simulink model "bpsk_receiver"  (R2020a)
settings: Solver=VariableStepAuto  StartTime=0.0  StopTime=10000/3.2e6  RelTol=1e-3
InitFcn:
  | setup_bpsk_receiver
undefined symbols (not defined in the file): AXI4, designMultirateFIR, fir_bbuf, Lite, tx_data, xlfda_numerator
libraries: xbsIndex_r4 x367, hdlsllib x15, dspmlti4 x8, xrbsSSR_Library x6, dspswit3 x4, dspsigops x2, commrandsrc3 x1, simulink x1
(part 2 of 4)

== system bpsk_receiver/Frame Synchronisation ==
  Reset : Inport
  Threshold : Inport  Port=2
  Valid In : Inport  Port=3
  Real In : Inport  Port=4
  Convert to AXI-Stream : Subsystem
  Frame Sync : Subsystem
  Valid Out : Outport  VectorParamsAs1DForOutWhenUnconnected=off
  Data Out : Outport  Port=2  VectorParamsAs1DForOutWhenUnconnected=off
  Last Out : Outport  Port=3  VectorParamsAs1DForOutWhenUnconnected=off
  Size : Outport  Port=4  VectorParamsAs1DForOutWhenUnconnected=off
  Count : Outport  Port=5  VectorParamsAs1DForOutWhenUnconnected=off
  wires:
  Convert to AXI-Stream/4(Size) -> Size/1
  Frame Sync/3(count) -> Count/1
  Convert to AXI-Stream/5(Reset) -> Frame Sync/5(Reset)
  Convert to AXI-Stream/3(Last Out) -> Last Out/1
  Convert to AXI-Stream/2(Valid Out) -> Valid Out/1
  Convert to AXI-Stream/1(Data Out) -> Data Out/1
  Frame Sync/2(Valid Out) -> Convert to AXI-Stream/2(Valid In)
  Frame Sync/1(Data Out) -> Convert to AXI-Stream/1(Data In)
  Reset/1 -> Frame Sync/4(reset_count)
  Valid In/1 -> Frame Sync/3(Valid In)
  Real In/1 -> Frame Sync/2(Data In)
  Threshold/1 -> Frame Sync/1(Threshold)

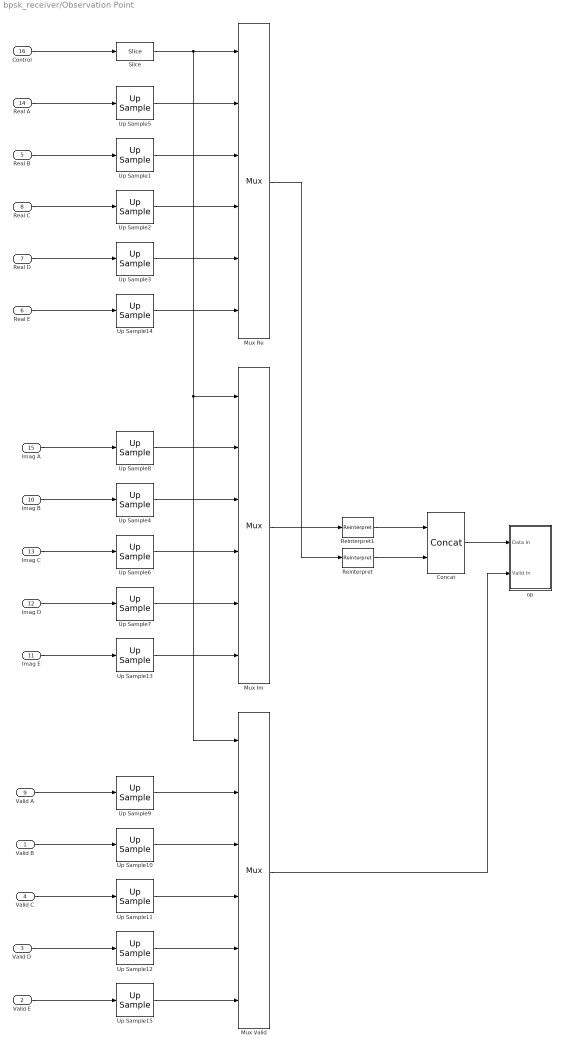
== system bpsk_receiver/Observation Point ==
  Valid B : Inport
  Valid E : Inport  Port=2
  Valid D : Inport  Port=3
  Valid C : Inport  Port=4
  Real B : Inport  Port=5
  Real E : Inport  Port=6
  Real D : Inport  Port=7
  Real C : Inport  Port=8
  Valid A : Inport  Port=9
  Imag B : Inport  Port=10
  Imag E : Inport  Port=11
  Imag D : Inport  Port=12
  Imag C : Inport  Port=13
  Real A : Inport  Port=14
  Imag A : Inport  Port=15
  Control : Inport  Port=16
  Concat : xbsIndex_r4/Concat  num_inputs=2  dbl_ovrd=off  block_type=concat
  Mux Im : xbsIndex_r4/Mux  inputs=5  en=off  latency=1  precision=Full  arith_type=Unsigned  n_bits=16  bin_pt=14  quantization=Truncate  overflow=Wrap  dbl_ovrd=off  block_type=mux
  Mux Re : xbsIndex_r4/Mux  inputs=5  en=off  latency=1  precision=Full  arith_type=Unsigned  n_bits=16  bin_pt=14  quantization=Truncate  overflow=Wrap  dbl_ovrd=off  block_type=mux
  Mux Valid : xbsIndex_r4/Mux  inputs=5  en=off  latency=1  precision=Full  arith_type=Unsigned  n_bits=16  bin_pt=14  quantization=Truncate  overflow=Wrap  dbl_ovrd=off  block_type=mux
  Reinterpret : xbsIndex_r4/Reinterpret  force_arith_type=on  arith_type=Unsigned  force_bin_pt=on  bin_pt=0  block_type=reinterpret
  Reinterpret1 : xbsIndex_r4/Reinterpret  force_arith_type=on  arith_type=Unsigned  force_bin_pt=on  bin_pt=0  block_type=reinterpret
  Slice : xbsIndex_r4/Slice  nbits=1  boolean_output=off  mode=Two Bit Locations  bit1=2  base1=LSB of Input  bit0=0  base0=LSB of Input  dbl_ovrd=off  block_type=slice
  Up Sample{1..2,4..6,8} (6 alike) : xbsIndex_r4/Up Sample  sample_ratio=64e6/3.2e6  copy_samples=on  en=off  latency=0  dbl_ovrd=off  block_type=usamp
  Up Sample10 : xbsIndex_r4/Up Sample  sample_ratio=64e6/3.2e6  copy_samples=off  en=off  latency=0  dbl_ovrd=off  block_type=usamp
  Up Sample11 : xbsIndex_r4/Up Sample  sample_ratio=64e6/3.2e6  copy_samples=off  en=off  latency=0  dbl_ovrd=off  block_type=usamp
  Up Sample12 : xbsIndex_r4/Up Sample  sample_ratio=64e6/12.8e6  copy_samples=off  en=off  latency=0  dbl_ovrd=off  block_type=usamp
  Up Sample{3,7,13..14} (4 alike) : xbsIndex_r4/Up Sample  sample_ratio=64e6/12.8e6  copy_samples=on  en=off  latency=0  dbl_ovrd=off  block_type=usamp
  Up Sample15 : xbsIndex_r4/Up Sample  sample_ratio=64e6/12.8e6  copy_samples=off  en=off  latency=0  dbl_ovrd=off  block_type=usamp
  Up Sample9 : xbsIndex_r4/Up Sample  sample_ratio=64e6/3.2e6  copy_samples=off  en=off  latency=0  dbl_ovrd=off  block_type=usamp
  op : Subsystem
  wires:
  Valid B/1 -> Up Sample10/1
  Up Sample10/1 -> Mux Valid/3
  Control/1 -> Slice/1
  Up Sample1/1 -> Mux Re/3
  Concat/1 -> op/1(Data In)
  Mux Re/1 -> Reinterpret/1
  Real B/1 -> Up Sample1/1
  Up Sample11/1 -> Mux Valid/4
  Up Sample2/1 -> Mux Re/4
  Mux Valid/1 -> op/2(Valid In)
  Up Sample3/1 -> Mux Re/5
  Up Sample6/1 -> Mux Im/4
  Up Sample12/1 -> Mux Valid/5
  Imag A/1 -> Up Sample8/1
  Real A/1 -> Up Sample5/1
  Reinterpret/1 -> Concat/2
  Up Sample7/1 -> Mux Im/5
  Reinterpret1/1 -> Concat/1
  Imag C/1 -> Up Sample6/1
  Up Sample5/1 -> Mux Re/2
  Up Sample4/1 -> Mux Im/3
  Up Sample8/1 -> Mux Im/2
  Mux Im/1 -> Reinterpret1/1
  Up Sample9/1 -> Mux Valid/2
  Valid A/1 -> Up Sample9/1
  Imag D/1 -> Up Sample7/1
  Valid D/1 -> Up Sample12/1
  Real D/1 -> Up Sample3/1
  Valid C/1 -> Up Sample11/1
  Valid E/1 -> Up Sample15/1
  Imag E/1 -> Up Sample13/1
  Real C/1 -> Up Sample2/1
  Imag B/1 -> Up Sample4/1
  Real E/1 -> Up Sample14/1
  Slice/1 -> Mux Valid/1, Mux Im/1, Mux Re/1
  Up Sample13/1 -> Mux Im/6
  Up Sample14/1 -> Mux Re/6
  Up Sample15/1 -> Mux Valid/6

== system bpsk_receiver/RRC Receive Filter ==
  Valid In : Inport
  Real In : Inport  Port=2
  Imag In : Inport  Port=3
  Convert : xbsIndex_r4/Convert  gui_display_data_type=Fixed-point  arith_type="Signed  (2's comp)"  n_bits=16  bin_pt=14  float_type=Single  exp_bits=8  fraction_bits=24  quantization=Truncate  overflow=Wrap  en=off  latency=0  pipeline=off  dbl_ovrd=off  block_type=convert
  Convert1 : xbsIndex_r4/Convert  gui_display_data_type=Fixed-point  arith_type="Signed  (2's comp)"  n_bits=16  bin_pt=14  float_type=Single  exp_bits=8  fraction_bits=24  quantization=Truncate  overflow=Wrap  en=off  latency=0  pipeline=off  dbl_ovrd=off  block_type=convert
  FDATool : xbsIndex_r4/FDATool  block_type=fdatool
      settings: infoedit=FDATool
  "FIR Compiler 7.2 " : xbsIndex_r4/FIR Compiler 7.2   coefficientvector=xlfda_numerator('FDATool')  coefficient_sets=1  coefficient_reload=off  filter_type=Decimation  rate_change_type=Integer  interpolation_rate=1  decimation_rate=4  zero_pack_factor=1  channel_sequence=Basic  number_channels=1  pattern_list='P4-0,P4-1,P4-2,P4-3,P4-4'  number_paths=2  ratespecification=Maximum_Possible  sampleperiod=1  hardwareoversamplingrate=1  coefficient_sign=Signed  quantization=Quantize_Only  coefficient_width=16  bestprecision=on  coefficient_fractional_bits=16  coefficient_structure=Inferred  output_rounding_mode=Full_Precision  output_width=33  filter_architecture=Systolic_Multiply_Accumulate  optimization_goal=Area  optimization_list='None'  data_buffer_type=Automatic  coefficient_buffer_type=Automatic  input_buffer_type=Automatic  output_buffer_type=Automatic  preference_for_other_storage=Automatic  multi_column_support=Automatic  columnconfig='6'  inter_column_pipe_length=4  data_has_tlast=Not_Required  m_data_has_tready=off  s_data_has_fifo=off  s_data_has_tuser=Not_Required  m_data_has_tuser=Not_Required  s_config_sync_mode=On_Vector  s_config_method=Single  num_reload_slots=1  has_aclken=off  has_aresetn=off  infoeditControl=ARESETn must be asserted for a minimum of 2 cycles  reset_data_vector=on  trim_axipin_name=on  simulation_type=hybrid_sim  simulation_model=sysgen:xfirv7_2_cmodel  data_path_portlist={ 's_axis_data_tdata', 'm_axis_data_tdata' }  passband_min=0.0  passband_max=0.5  stopband_min=0.5  stopband_max=1.0  filter_selection=1  gui_behaviour='Sysgen_GUI'  data_sign=Signed  data_width=16  data_fractional_bits=0  data_tuser_width=1  wrapper_available=true  ip_wrap_arbitrary_binary_point=true  ip_name=FIR Compiler  ip_version=7.2  dsptool_ready=true  ipcore_usecache=true  ipcore_useipmodelcache=true  port_translation_map={ 'aclken' => 'en', 'aresetn' => 'rst' }  run_core_at_system_period=true  ipcore_xco_need_fpga_part=true  block_type=fir_compiler_v7_2
      settings: infoedit=Maximum Possible : Maximizes oversampling rate. Abstracted input handshake (no s_data_tvalid) and automatic rate propagation.<br>Hardware Oversampling Rate : Specifies oversampling rate relative to the input sample period. Abstracted input handshake (no s_data_tvalid) and automatic rate propagation.<br>Input/Output Sample Period : Specifies absolute oversampling rate. No input handshake abstraction (exposes s_data_tvalid) and no rate propagation.
  Terminator2 : Terminator
  Terminator4 : Terminator
  Valid Out : Outport  VectorParamsAs1DForOutWhenUnconnected=off
  Real Out : Outport  Port=2  VectorParamsAs1DForOutWhenUnconnected=off
  Imag Out : Outport  Port=3  VectorParamsAs1DForOutWhenUnconnected=off
  wires:
  "FIR Compiler 7.2 "/2 -> Valid Out/1
  "FIR Compiler 7.2 "/4 -> Convert1/1
  Imag In/1 -> "FIR Compiler 7.2 "/2
  "FIR Compiler 7.2 "/1 -> Terminator2/1
  Real In/1 -> "FIR Compiler 7.2 "/1
  Convert/1 -> Real Out/1
  "FIR Compiler 7.2 "/3 -> Convert/1
  Convert1/1 -> Imag Out/1
  Valid In/1 -> Terminator4/1

== system bpsk_receiver/SSR Halfband Lowpass Decimator ==
  Valid In : Inport
  Real In : Inport  Port=2
  Imag In : Inport  Port=3
  Convert : xbsIndex_r4/Convert  gui_display_data_type=Fixed-point  arith_type="Signed  (2's comp)"  n_bits=16  bin_pt=14  float_type=Single  exp_bits=8  fraction_bits=24  quantization="Round  (unbiased: +/- Inf)"  overflow=Saturate  en=off  latency=0  pipeline=off  dbl_ovrd=off  block_type=convert
  Convert1 : xbsIndex_r4/Convert  gui_display_data_type=Fixed-point  arith_type="Signed  (2's comp)"  n_bits=16  bin_pt=14  float_type=Single  exp_bits=8  fraction_bits=24  quantization="Round  (unbiased: +/- Inf)"  overflow=Saturate  en=off  latency=0  pipeline=off  dbl_ovrd=off  block_type=convert
  FDATool : xbsIndex_r4/FDATool  block_type=fdatool
      settings: infoedit=FDATool
  Terminator1 : Terminator
  Terminator2 : Terminator
  Vector FIR Im : xrbsSSR_Library/Vector FIR  coefficientvector=xlfda_numerator('FDATool')/(max(xlfda_numerator('FDATool'))*2)  coefficient_sets=1  coeffsets_prev=1  coefficient_reload=off  filter_type=Decimation  filter_prev=Decimation  interpolation_rate=2  interpolation_prev=2  rate_change_type=Integer  decimation_rate=2  decimation_prev=2  zero_pack_factor=2  channel_sequence=Basic  number_channels=1  pattern_list='P4-0,P4-1,P4-2,P4-3,P4-4'  number_paths=1  sg_ssr=2  coefficient_sign=Signed  quantization=Quantize_Only  coefficient_width=16  bestprecision=off  coefficient_fractional_bits=14  coefficient_structure=Inferred  output_rounding_mode=Full_Precision  output_width=24  filter_architecture=Systolic_Multiply_Accumulate  optimization_goal=Area  optimization_list='None'  data_buffer_type=Automatic  coefficient_buffer_type=Automatic  input_buffer_type=Automatic  output_buffer_type=Automatic  preference_for_other_storage=Automatic  multi_column_support=Automatic  columnconfig='11'  inter_column_pipe_length=4  data_has_tlast=Not_Required  m_data_has_tready=off  s_data_has_fifo=off  s_data_has_tuser=Not_Required  m_data_has_tuser=Not_Required  s_config_sync_mode=On_Vector  s_config_method=Single  num_reload_slots=1  has_aclken=off  has_aresetn=off  infoeditControl=ARESETn must be asserted for a minimum of 2 cycles  reset_data_vector=on  simulation_type=xsim  simulation_model=sysgen:xfirv7_2_cmodel  data_path_portlist={ 's_axis_data_tdata', 'm_axis_data_tdata' }  passband_min=0.0  passband_max=0.5  stopband_min=0.5  stopband_max=1.0  filter_selection=1  gui_behaviour=1  data_sign=Signed  data_width=16  data_fractional_bits=0  data_tuser_width='11'  wrapper_available=true  ip_wrap_arbitrary_binary_point=true  ip_name=FIR Compiler  ip_version=7.2  dsptool_ready=true  ipcore_usecache=true  ipcore_useipmodelcache=true  port_translation_map={ 'aclken' => 'en', 'aresetn' => 'rst' }  run_core_at_system_period=true  ipcore_xco_need_fpga_part=true  ipcore_fpga_part=[]  block_type=fir_compiler_v7_2_ssr  sg_ssr_name=vect_FIR  sg_ssr_prev=2
      settings: SourceProductName=Xilinx SSR Blockset
  Vector FIR Re : xrbsSSR_Library/Vector FIR  coefficientvector=xlfda_numerator('FDATool')/(max(xlfda_numerator('FDATool'))*2)  coefficient_sets=1  coeffsets_prev=1  coefficient_reload=off  filter_type=Decimation  filter_prev=Decimation  interpolation_rate=2  interpolation_prev=2  rate_change_type=Integer  decimation_rate=2  decimation_prev=2  zero_pack_factor=2  channel_sequence=Basic  number_channels=1  pattern_list='P4-0,P4-1,P4-2,P4-3,P4-4'  number_paths=1  sg_ssr=2  coefficient_sign=Signed  quantization=Quantize_Only  coefficient_width=16  bestprecision=off  coefficient_fractional_bits=14  coefficient_structure=Inferred  output_rounding_mode=Full_Precision  output_width=24  filter_architecture=Systolic_Multiply_Accumulate  optimization_goal=Area  optimization_list='None'  data_buffer_type=Automatic  coefficient_buffer_type=Automatic  input_buffer_type=Automatic  output_buffer_type=Automatic  preference_for_other_storage=Automatic  multi_column_support=Automatic  columnconfig='11'  inter_column_pipe_length=4  data_has_tlast=Not_Required  m_data_has_tready=off  s_data_has_fifo=off  s_data_has_tuser=Not_Required  m_data_has_tuser=Not_Required  s_config_sync_mode=On_Vector  s_config_method=Single  num_reload_slots=1  has_aclken=off  has_aresetn=off  infoeditControl=ARESETn must be asserted for a minimum of 2 cycles  reset_data_vector=on  simulation_type=xsim  simulation_model=sysgen:xfirv7_2_cmodel  data_path_portlist={ 's_axis_data_tdata', 'm_axis_data_tdata' }  passband_min=0.0  passband_max=0.5  stopband_min=0.5  stopband_max=1.0  filter_selection=1  gui_behaviour=1  data_sign=Signed  data_width=16  data_fractional_bits=0  data_tuser_width='11'  wrapper_available=true  ip_wrap_arbitrary_binary_point=true  ip_name=FIR Compiler  ip_version=7.2  dsptool_ready=true  ipcore_usecache=true  ipcore_useipmodelcache=true  port_translation_map={ 'aclken' => 'en', 'aresetn' => 'rst' }  run_core_at_system_period=true  ipcore_xco_need_fpga_part=true  ipcore_fpga_part=[]  block_type=fir_compiler_v7_2_ssr  sg_ssr_name=vect_FIR  sg_ssr_prev=2
      settings: SourceProductName=Xilinx SSR Blockset
  Valid Out : Outport  VectorParamsAs1DForOutWhenUnconnected=off
  Real Out : Outport  Port=2  VectorParamsAs1DForOutWhenUnconnected=off
  Imag Out : Outport  Port=3  VectorParamsAs1DForOutWhenUnconnected=off
  Ready Out : Outport  Port=4  VectorParamsAs1DForOutWhenUnconnected=off
  wires:
  Convert1/1 -> Imag Out/1
  Convert/1 -> Real Out/1
  Vector FIR Im/2 -> Terminator2/1
  Vector FIR Re/1 -> Ready Out/1
  Vector FIR Im/1 -> Terminator1/1
  Vector FIR Im/3 -> Convert1/1
  Vector FIR Re/3 -> Convert/1
  Real In/1 -> Vector FIR Re/2
  Vector FIR Re/2 -> Valid Out/1
  Valid In/1 -> Vector FIR Re/1, Vector FIR Im/1
  Imag In/1 -> Vector FIR Im/2

== system bpsk_receiver/Time Synchronisation ==
  Reset : Inport
  Valid In : Inport  Port=2
  Real In : Inport  Port=3
  Imag In : Inport  Port=4
  Loop Filter : Subsystem  mask{T=1/100e3, d=1/sqrt(2), Kp=3.2, Bn=100e3*0.05, Ko=1}
      mask prompts: T "Sampling Period:"; d "Damping Ratio:"; Kp "Phase Detector Gain:"; Bn "Noise Bandwidth:"; Ko "Oscillator Gain:"
      mask init:
      | n = (Bn*T)/(d+1/(4*d));
      | 
      | K1 = ((4*d*n)/(1+2*d*n+n^2))/(Ko*Kp);
      | 
      | K2 = ((4*n^2)/(1+2*d*n+n^2))/(Ko*Kp);
      | 
      | %K1 = (4*d*n)/(Ko*Kp);
      | 
      | %K2 = (4*(n^2))/(Ko*Kp);
      mask DialogControl DescGroupVar Prompt: Loop Filter
      mask DialogControl DescTextVar Prompt: A simplified loop filter.
      mask DialogControl ParameterGroupVar Prompt: Main
  NCC : Subsystem  mask{r=32, f=58}
      mask prompts: r "Symbol Oversample Factor:"; f "Fractional Bits:"
      mask init:
      | n = ceil(log2(r))+1;
      mask DialogControl DescGroupVar Prompt: Numerically Controlled Clock (NCC)
      mask DialogControl DescTextVar Prompt: The NCC block contains an accumulator that increments by one each clock cycle. The wordlength of the accumulator is determined by the symbol oversampling factor. Once the maximum value of the accumulator is reached, the accumulation starts again. The error signal can be used to increase or decrease the rate of accumulation. When the accumulator wraps around, a binary high is released from the strobe port.
      mask DialogControl ParameterGroupVar Prompt: Main
  Terminator : Terminator
  Timing Error Detector : Subsystem
  Valid Out : Outport  VectorParamsAs1DForOutWhenUnconnected=off
  Real Out : Outport  Port=2  VectorParamsAs1DForOutWhenUnconnected=off
  Imag Out : Outport  Port=3  VectorParamsAs1DForOutWhenUnconnected=off
  wires:
  Valid In/1 -> Terminator/1
  Real In/1 -> Timing Error Detector/1(Real In), Loop Filter/1(Real In)
  Loop Filter/4(Error Out) -> NCC/1(Error)
  Timing Error Detector/1(Error) -> Loop Filter/3(Signal In)
  Imag In/1 -> Loop Filter/2(Imag In), Timing Error Detector/2(Imag In)
  Loop Filter/3(Valid Out) -> Valid Out/1
  Loop Filter/1(Real Out) -> Real Out/1
  Loop Filter/2(Imag Out) -> Imag Out/1
  NCC/1(Strobe) -> Loop Filter/4(Valid In)
  Reset/1 -> Loop Filter/5(Reset)

== system bpsk_receiver/AXI-Stream Master Interface/Rising Edge Detector Enable ==
  Input : Inport
  Inverter2 : xbsIndex_r4/Inverter  en=off  latency=0  dbl_ovrd=off  block_type=inv
  Logical3 : xbsIndex_r4/Logical  logical_function=AND  inputs=2  en=off  latency=0  precision=Full  arith_type=Unsigned  n_bits=16  bin_pt=0  align_bp=on  dbl_ovrd=off  block_type=logical
  Register1 : xbsIndex_r4/Register  init=0  rst=off  en=off  dbl_ovrd=off  block_type=register
  Output : Outport  VectorParamsAs1DForOutWhenUnconnected=off
  wires:
  Input/1 -> Logical3/2, Inverter2/1
  Inverter2/1 -> Register1/1
  Logical3/1 -> Output/1
  Register1/1 -> Logical3/1

== system bpsk_receiver/AXI-Stream Master Interface/Rising Edge Detector Last ==
  Input : Inport
  Inverter2 : xbsIndex_r4/Inverter  en=off  latency=0  dbl_ovrd=off  block_type=inv
  Logical3 : xbsIndex_r4/Logical  logical_function=AND  inputs=2  en=off  latency=0  precision=Full  arith_type=Unsigned  n_bits=16  bin_pt=0  align_bp=on  dbl_ovrd=off  block_type=logical
  Register1 : xbsIndex_r4/Register  init=0  rst=off  en=off  dbl_ovrd=off  block_type=register
  Output : Outport  VectorParamsAs1DForOutWhenUnconnected=off
  wires:
  Register1/1 -> Logical3/1
  Logical3/1 -> Output/1
  Inverter2/1 -> Register1/1
  Input/1 -> Inverter2/1, Logical3/2

== system bpsk_receiver/BPSK System/BPSK TX Generation ==
  Enable : Inport
  Bernoulli Binary Generator : commrandsrc3/Bernoulli Binary Generator  ProbabilityOfZero=0.5  SeedSource=Auto  Seed=0  SampleTime=1/100e3  SamplesPerFrame=1  OutputDataType=double  SimulateUsing=Interpreted execution
  CIC Interpolation : dspmlti4/CIC Interpolation  filtFrom=Dialog parameters  filtobj=Hm_interp  ftype=Interpolator  R=320  M=1  N=5  filterInternals=Full precision  BPS=[16 16 16 16]  FLPS=0  outputWordLength=32  outputFracLength=0  launchFVT=off  framing=Allow multirate processing  OutputFrames=off
      settings: SourceProductBaseCode=DS
  Constant : Constant  SampleTime=1/12.5e3
  DBPSK Modulator : Subsystem
  DMA Read : Subsystem
  Data Type Conversion2 : DataTypeConversion  OutDataTypeStr=fixdt(1,16,14)
  FDATool : xbsIndex_r4/FDATool  block_type=fdatool
      settings: infoedit=FDATool
  FIR Interpolation : dspmlti4/FIR Interpolation  FilterSource=Dialog parameters  PrivateCoeffs=0  h=xlfda_numerator('FDATool')*4  L=4  FilterObject=xlfda_numerator('FDATool')/(max(xlfda_numerator('FDATool')))  framing=Allow multirate processing  outputBufInitCond=0  roundingMode=Floor  overflowMode=off  firstCoeffMode=Binary point scaling  firstCoeffWordLength=16  firstCoeffFracLength=14  firstCoeffDataTypeStr=fixdt(1,16,14)  firstCoeffMin=[]  firstCoeffMax=[]  firstCoeffLastDataTypeStr=fixdt(1,16,14)  outputDataTypeStr=Inherit: Same as accumulator  outputMin=[]  outputMax=[]  outputLastDataTypeStr=Inherit: Same as accumulator
  Multiply : Gain  Gain=fi(0.8192, 1, 16, 14)  ParamDataTypeStr=fixdt(1,16,15)  OutDataTypeStr=fixdt(1,16,14)
  Multiport Switch : MultiPortSwitch  DataPortOrder=Zero-based contiguous  Inputs=2  zeroidx=on
  Shift Arithmetic : ArithShift  BitShiftNumber=33  BitShiftDirection=Right
  Terminator1 : Terminator
  BPSK : Outport  VectorParamsAs1DForOutWhenUnconnected=off
  wires:
  CIC Interpolation/1 -> Shift Arithmetic/1
  FIR Interpolation/1 -> Data Type Conversion2/1
  Bernoulli Binary Generator/1 -> Multiport Switch/2
  DMA Read/2(tvalid) -> Multiport Switch/1
  DMA Read/1(tdata) -> Multiport Switch/3
  DMA Read/3(tlast) -> Terminator1/1
  Enable/1 -> DMA Read/1(enable)
  Constant/1 -> DMA Read/2(tready)
  Multiport Switch/1 -> DBPSK Modulator/1(Input)
  Multiply/1 -> BPSK/1
  DBPSK Modulator/1(Output) -> FIR Interpolation/1
  Data Type Conversion2/1 -> CIC Interpolation/1
  Shift Arithmetic/1 -> Multiply/1

== system bpsk_receiver/BPSK System/RF-ADC ==
  Data In : Inport
  Decimation Filter : Subsystem  mask{decim=8x}
      mask prompts: decim "Decimation Factor:"
      mask init:
      | fir0 = dsp.FIRDecimator('DecimationFactor', 2,...
      |                            'CoefficientsDataType', 'Custom',...
      |                            'CustomCoefficientsDataType', numerictype([], 16, 14),...
      |                            'FullPrecisionOverride', false,...
      |                            'OutputDataType', 'Custom',...
      |                            'CustomOutputDataType', numerictype([], 16, 14),...
      |                            'Numerator', [-6, 0 54, 0, -254, 0, 1230, 2048, 1230, 0, -254, 0, 54, 0, -6]/(2048*2));
      | fir1 = dsp.FIRDecimator('DecimationFactor', 2,...
      |                            'CoefficientsDataType', 'Custom',...
      |                            'CustomCoefficientsDataType', numerictype([], 16, 14),...
      |                            'FullPrecisionOverride', false,...
      |                            'OutputDataType', 'Custom',...
      |                            'CustomOutputDataType', numerictype([], 16, 14),...
      |                            'Numerator', [-12, 0, 84, 0, -337, 0, 1008, 0, -2693, 0, 10142, 16384, 10142, 0, -2693, 0, 1008, 0, -337, 0, 84, 0 ,-12]/(16384*2));
      | fir2 = dsp.FIRDecimator('DecimationFactor', 2,...
      |                            'CoefficientsDataType', 'Custom',...
      |                            'CustomCoefficientsDataType', numerictype([], 16, 14),...
      |                            'FullPrecisionOverride', false,...
      |                            'OutputDataType', 'Custom',...
      |                            'CustomOutputDataType', numerictype([], 16, 14),...
      |                            'Numerator', [5, 0, -17, 0, 44, 0, -96, 0, 187, 0, -335, 0, 565, 0, -906, 0, 1401, 0, -2112, 0, 3145, 0, -4723, 0, 7415, 0, -13331, 0, 41526, 65536, 41526, 0, -13331, 0, 7415, 0, -4723, 0, 3145, 0, -2112, 0, 1401, 0, -906, 0, 565, 0, -335, 0, 187, 0, -96, 0, 44, 0, -17, 0, 5]/(65536));
      | switch get_param(gcb, 'decim')
      |     case '1x'
      |         if ~strcmp(get_param([gcb, '/FIR 0'], 'Commented'), 'through')
      |             set_param([gcb, '/FIR 0'],'Commented','through');
      |         end
      |         
      |         if ~strcmp(get_param([gcb, '/FIR 1'], 'Commented'), 'through')
      |             set_param([gcb, '/FIR 1'],'Commented','through');
      |         end
      |         
      |         if ~strcmp(get_param([gcb, '/FIR 2'], 'Commented'), 'through')
      |             set_param([gcb, '/FIR 2'],'Commented','through');
      |         end
      |             
      |     case '2x'
      |         if ~strcmp(get_param([gcb, '/FIR 0'], 'Commented'), 'through')
      |             set_param([gcb, '/FIR 0'],'Commented','through');
      |         end
      |         
      |         if ~strcmp(get_param([gcb, '/FIR 1'], 'Commented'), 'through')
      |             set_param([gcb, '/FIR 1'],'Commented','through');
      |         end
      |         
      |         if ~strcmp(get_param([gcb, '/FIR 2'], 'Commented'), 'off')
      |             set_param([gcb, '/FIR 2'],'Commented','off');
      |         end
      | 
      |     case '4x'
      |         if ~strcmp(get_param([gcb, '/FIR 0'], 'Commented'), 'through')
      |             set_param([gcb, '/FIR 0'],'Commented','through');
      |         end
      |         
      |         if ~strcmp(get_param([gcb, '/FIR 1'], 'Commented'), 'off')
      |             set_param([gcb, '/FIR 1'],'Commented','off');
      |         end
      |         
      |         if ~strcmp(get_param([gcb, '/FIR 2'], 'Commented'), 'off')
      |             set_param([gcb, '/FIR 2'],'Commented','off');
      |         end
      |         
      |     case '8x'
      |         if ~strcmp(get_param([gcb, '/FIR 0'], 'Commented'), 'off')
      |             set_param([gcb, '/FIR 0'],'Commented','off');
      |         end
      |         
      |         if ~strcmp(get_param([gcb, '/FIR 1'], 'Commented'), 'off')
      |             set_param([gcb, '/FIR 1'],'Commented','off');
      |         end
      |         
      |         if ~strcmp(get_param([gcb, '/FIR 2'], 'Commented'), 'off')
      |             set_param([gcb, '/FIR 2'],'Commented','off');
      |         end
      | 
      | end
      mask TypeOptions decim: 1x | 2x | 4x | 8x
      mask DialogControl DescGroupVar Prompt: RF-DAC Interpolation Filter
      mask DialogControl DescTextVar Prompt: This block simulates the RF-DAC interpolation stage using the same coefficients stored in the interpolation filters.
      mask DialogControl ParameterGroupVar Prompt: Main
  NCO and Mixer : Subsystem
  RF-ADC : Subsystem
  Data Out : Outport  VectorParamsAs1DForOutWhenUnconnected=off
  wires:
  NCO and Mixer/1(Data Out) -> Decimation Filter/1(Data In)
  RF-ADC/1(Data Out) -> NCO and Mixer/1(Data In)
  Data In/1 -> RF-ADC/1(Data In)
  Decimation Filter/1(Data Out) -> Data Out/1

== system bpsk_receiver/BPSK System/RF-DAC ==
  note: Not Ready
  Data In : Inport
  Coarse Delay : Subsystem
  Interpolation Filter : Subsystem  mask{interp=8x}
      mask prompts: interp "Interpolation Factor:"
      mask init:
      | fir0 = dsp.FIRInterpolator('InterpolationFactor', 2,...
      |                            'CoefficientsDataType', 'Custom',...
      |                            'CustomCoefficientsDataType', numerictype([], 16, 14),...
      |                            'FullPrecisionOverride', false,...
      |                            'OutputDataType', 'Custom',...
      |                            'CustomOutputDataType', numerictype([], 16, 14),...
      |                            'Numerator', [-6, 0 54, 0, -254, 0, 1230, 2048, 1230, 0, -254, 0, 54, 0, -6]/(2048));
      | fir1 = dsp.FIRInterpolator('InterpolationFactor', 2,...
      |                            'CoefficientsDataType', 'Custom',...
      |                            'CustomCoefficientsDataType', numerictype([], 16, 14),...
      |                            'FullPrecisionOverride', false,...
      |                            'OutputDataType', 'Custom',...
      |                            'CustomOutputDataType', numerictype([], 16, 14),...
      |                            'Numerator', [-12, 0, 84, 0, -337, 0, 1008, 0, -2693, 0, 10142, 16384, 10142, 0, -2693, 0, 1008, 0, -337, 0, 84, 0 ,-12]/(16384));
      | fir2 = dsp.FIRInterpolator('InterpolationFactor', 2,...
      |                            'CoefficientsDataType', 'Custom',...
      |                            'CustomCoefficientsDataType', numerictype([], 16, 14),...
      |                            'FullPrecisionOverride', false,...
      |                            'OutputDataType', 'Custom',...
      |                            'CustomOutputDataType', numerictype([], 16, 14),...
      |                            'Numerator', [5, 0, -17, 0, 44, 0, -96, 0, 187, 0, -335, 0, 565, 0, -906, 0, 1401, 0, -2112, 0, 3145, 0, -4723, 0, 7415, 0, -13331, 0, 41526, 65536, 41526, 0, -13331, 0, 7415, 0, -4723, 0, 3145, 0, -2112, 0, 1401, 0, -906, 0, 565, 0, -335, 0, 187, 0, -96, 0, 44, 0, -17, 0, 5]/(65536));
      | switch get_param(gcb, 'interp')
      |     case '1x'
      |         if ~strcmp(get_param([gcb, '/FIR 0'], 'Commented'), 'through')
      |             set_param([gcb, '/FIR 0'],'Commented','through');
      |         end
      |         
      |         if ~strcmp(get_param([gcb, '/FIR 1'], 'Commented'), 'through')
      |             set_param([gcb, '/FIR 1'],'Commented','through');
      |         end
      |         
      |         if ~strcmp(get_param([gcb, '/FIR 2'], 'Commented'), 'through')
      |             set_param([gcb, '/FIR 2'],'Commented','through');
      |         end
      |             
      |     case '2x'
      |         if ~strcmp(get_param([gcb, '/FIR 0'], 'Commented'), 'through')
      |             set_param([gcb, '/FIR 0'],'Commented','through');
      |         end
      |         
      |         if ~strcmp(get_param([gcb, '/FIR 1'], 'Commented'), 'through')
      |             set_param([gcb, '/FIR 1'],'Commented','through');
      |         end
      |         
      |         if ~strcmp(get_param([gcb, '/FIR 2'], 'Commented'), 'off')
      |             set_param([gcb, '/FIR 2'],'Commented','off');
      |         end
      | 
      |     case '4x'
      |         if ~strcmp(get_param([gcb, '/FIR 0'], 'Commented'), 'through')
      |             set_param([gcb, '/FIR 0'],'Commented','through');
      |         end
      |         
      |         if ~strcmp(get_param([gcb, '/FIR 1'], 'Commented'), 'off')
      |             set_param([gcb, '/FIR 1'],'Commented','off');
      |         end
      |         
      |         if ~strcmp(get_param([gcb, '/FIR 2'], 'Commented'), 'off')
      |             set_param([gcb, '/FIR 2'],'Commented','off');
      |         end
      |         
      |     case '8x'
      |         if ~strcmp(get_param([gcb, '/FIR 0'], 'Commented'), 'off')
      |             set_param([gcb, '/FIR 0'],'Commented','off');
      |         end
      |         
      |         if ~strcmp(get_param([gcb, '/FIR 1'], 'Commented'), 'off')
      |             set_param([gcb, '/FIR 1'],'Commented','off');
      |         end
      |         
      |         if ~strcmp(get_param([gcb, '/FIR 2'], 'Commented'), 'off')
      |             set_param([gcb, '/FIR 2'],'Commented','off');
      |         end
      | 
      | end
      mask TypeOptions interp: 1x | 2x | 4x | 8x
      mask DialogControl DescGroupVar Prompt: RF-DAC Interpolation Filter
      mask DialogControl DescTextVar Prompt: This block simulates the RF-DAC interpolation stage using the same coefficients stored in the interpolation filters.
      mask DialogControl ParameterGroupVar Prompt: Main
  NCO and Mixer : Subsystem
  Output Filter : Subsystem
  QMC Gain & Phase : Subsystem
  QMC Threshold : Subsystem
  RF-DAC : Subsystem
  Data Out : Outport  VectorParamsAs1DForOutWhenUnconnected=off
  wires:
  RF-DAC/1(Data Out) -> Data Out/1
  QMC Threshold/1(Data Out) -> RF-DAC/1(Data In)
  Output Filter/1(Data Out) -> QMC Threshold/1(Data In)
  Coarse Delay/1(Data Out) -> Output Filter/1(Data In)
  QMC Gain & Phase/1(Data Out) -> Coarse Delay/1(Data In)
  Data In/1 -> Interpolation Filter/1(Data In)
  NCO and Mixer/1(Data Out) -> QMC Gain & Phase/1(Data In)
  Interpolation Filter/1(Data Out) -> NCO and Mixer/1(Data In)

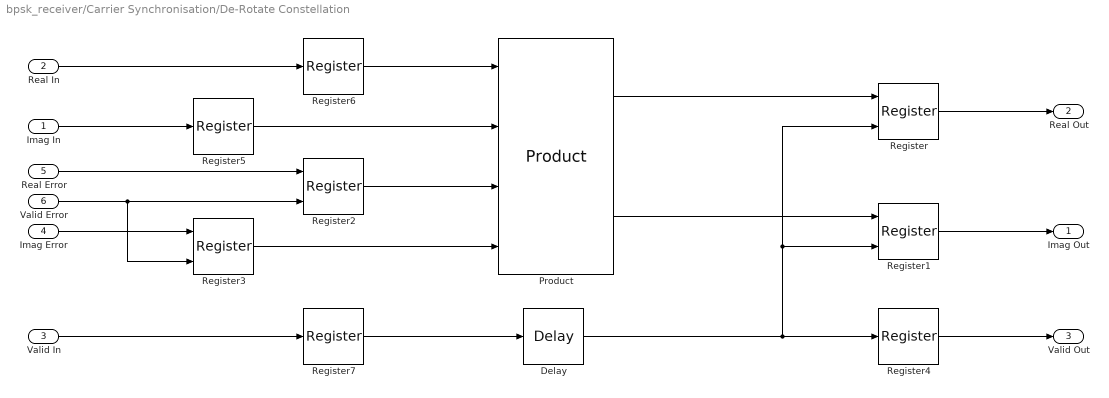
== system bpsk_receiver/Carrier Synchronisation/De-Rotate Constellation ==
  Imag In : Inport
  Real In : Inport  Port=2
  Valid In : Inport  Port=3
  Imag Error : Inport  Port=4
  Real Error : Inport  Port=5
  Valid Error : Inport  Port=6
  Delay : xbsIndex_r4/Delay  rst=off  infoeditControl=Selection of Reset will increase slice count due to use of real FFs and instead of SRLs  en=off  latency=4  reg_retiming=off  dbl_ovrd=off  block_type=delay
  Product : xbsIndex_r4/Product  complex_multiplier=on  optimizegoal=Performance  simulation_type=fast_sim  simulation_model=sysgen:product_macro  block_type=product_macro
  Register{,1..3} (4 alike) : xbsIndex_r4/Register  init=0  rst=off  en=on  dbl_ovrd=off  block_type=register
  Register{4..7} (4 alike) : xbsIndex_r4/Register  init=0  rst=off  en=off  dbl_ovrd=off  block_type=register
  Imag Out : Outport  VectorParamsAs1DForOutWhenUnconnected=off
  Real Out : Outport  Port=2  VectorParamsAs1DForOutWhenUnconnected=off
  Valid Out : Outport  Port=3  VectorParamsAs1DForOutWhenUnconnected=off
  wires:
  Register/1 -> Real Out/1
  Register1/1 -> Imag Out/1
  Valid In/1 -> Register7/1
  Imag Error/1 -> Register3/1
  Register4/1 -> Valid Out/1
  Register7/1 -> Delay/1
  Real Error/1 -> Register2/1
  Imag In/1 -> Register5/1
  Real In/1 -> Register6/1
  Valid Error/1 -> Register3/2, Register2/2
  Delay/1 -> Register/2, Register1/2, Register4/1
  Register6/1 -> Product/1
  Register5/1 -> Product/2
  Register2/1 -> Product/3
  Register3/1 -> Product/4
  Product/1 -> Register/1
  Product/2 -> Register1/1

== system bpsk_receiver/Carrier Synchronisation/Generate Angle Error ==
  Imag In : Inport
  Real In : Inport  Port=2
  Valid In : Inport  Port=3
  Circular CORDIC : Subsystem
  Delay : xbsIndex_r4/Delay  rst=off  infoeditControl=Selection of Reset will increase slice count due to use of real FFs and instead of SRLs  en=off  latency=8  reg_retiming=off  dbl_ovrd=off  block_type=delay
  Register : xbsIndex_r4/Register  init=0  rst=off  en=on  dbl_ovrd=off  block_type=register
  Register1 : xbsIndex_r4/Register  init=0  rst=off  en=on  dbl_ovrd=off  block_type=register
  Register3 : xbsIndex_r4/Register  init=0  rst=off  en=off  dbl_ovrd=off  block_type=register
  Angle : Outport  VectorParamsAs1DForOutWhenUnconnected=off
  Valid Out : Outport  Port=2  VectorParamsAs1DForOutWhenUnconnected=off
  wires:
  Delay/1 -> Valid Out/1
  Circular CORDIC/1(Angle) -> Angle/1
  Valid In/1 -> Register3/1, Register/2, Register1/2
  Real In/1 -> Register/1
  Imag In/1 -> Register1/1
  Register1/1 -> Circular CORDIC/1(Imag In)
  Register3/1 -> Delay/1
  Register/1 -> Circular CORDIC/2(Real In)

== system bpsk_receiver/Carrier Synchronisation/Generate NCO ==
  Angle : Inport
  Valid In : Inport  Port=2
  Reset : Inport  Port=3
  Loop Filter : Subsystem  mask{T=1/(100e3*32), d=0.707, Kp=1, Bn=0.04*(100e3*32), Ko=1}
      mask prompts: T "Sampling Period:"; d "Damping Ratio:"; Kp "Phase Detector Gain:"; Bn "Noise Bandwidth:"; Ko "Oscillator Gain:"
      mask init:
      | n = (Bn*T)/(d+1/(4*d));
      | 
      | %K1 = ((4*d*n)/(1+2*d*n+n^2))/(Ko*Kp);
      | 
      | %K2 = ((4*n^2)/(1+2*d*n+n^2))/(Ko*Kp);
      | 
      | K1 = (4*d*n)/(Ko*Kp);
      | 
      | K2 = (4*(n^2))/(Ko*Kp);
  NCO : Subsystem  mask(NCO){n=8, b=32-8}
      mask prompts: n "Number of integer_bits"; b "Number of fractional bits"
      mask help:
      | Numerically Controller Oscillator.
      |
      | Integrates the phase error and generates cosine and negative sign outputs.
      mask init:
      | k_n = ceil(log2((2^n)/(2*pi)));
      mask DialogControl Container3 Prompt: Accumulator
  Imag Out : Outport  VectorParamsAs1DForOutWhenUnconnected=off
  Real Out : Outport  Port=2  VectorParamsAs1DForOutWhenUnconnected=off
  Valid Out : Outport  Port=3  VectorParamsAs1DForOutWhenUnconnected=off
  wires:
  Reset/1 -> Loop Filter/3(Reset)
  NCO/1(Cos) -> Real Out/1
  NCO/2(Neg Sin) -> Imag Out/1
  Loop Filter/2(Valid) -> NCO/2(En_in)
  Loop Filter/1(Error) -> NCO/1(Step Size)
  Valid In/1 -> Loop Filter/2(Strobe)
  Angle/1 -> Loop Filter/1(Signal)
  NCO/3(En_out) -> Valid Out/1

== system bpsk_receiver/Coarse Frequency Synchronisation/Apply Frequency Offset Correction ==
  Imag In : Inport
  Real In : Inport  Port=2
  cos : Inport  Port=3
  sin : Inport  Port=4
  Convert : xbsIndex_r4/Convert  gui_display_data_type=Fixed-point  arith_type="Signed  (2's comp)"  n_bits=16  bin_pt=14  float_type=Single  exp_bits=8  fraction_bits=24  quantization=Truncate  overflow=Saturate  en=off  latency=0  pipeline=off  dbl_ovrd=off  block_type=convert
  Convert1 : xbsIndex_r4/Convert  gui_display_data_type=Fixed-point  arith_type="Signed  (2's comp)"  n_bits=16  bin_pt=14  float_type=Single  exp_bits=8  fraction_bits=24  quantization=Truncate  overflow=Saturate  en=off  latency=0  pipeline=off  dbl_ovrd=off  block_type=convert
  Product : xbsIndex_r4/Product  complex_multiplier=on  optimizegoal=Performance  simulation_type=fast_sim  simulation_model=sysgen:product_macro  block_type=product_macro
  Imag Out : Outport  VectorParamsAs1DForOutWhenUnconnected=off
  Real Out : Outport  Port=2  VectorParamsAs1DForOutWhenUnconnected=off
  wires:
  Product/1 -> Convert/1
  Product/2 -> Convert1/1
  Imag In/1 -> Product/2
  Real In/1 -> Product/1
  cos/1 -> Product/3
  sin/1 -> Product/4
  Convert/1 -> Real Out/1
  Convert1/1 -> Imag Out/1

== system bpsk_receiver/Coarse Frequency Synchronisation/Get Frequency Offset ==
  Mag In : Inport
  SoF : Inport  Port=2
  Constant : xbsIndex_r4/Constant  const=1023  gui_display_data_type=Fixed-point  arith_type=Unsigned  n_bits=10  bin_pt=0  preci_type=Single  exp_width=8  frac_width=24  explicit_period=off  period=1  equ=P=C  opselect=C  inp2=PCIN>>17  opr=+  inp1=P  carry=CIN  dbl_ovrd=off  block_type=constant
  Counter : xbsIndex_r4/Counter  cnt_type=Count Limited  cnt_to=1023  operation=Up  start_count=0  cnt_by_val=1  arith_type=Unsigned  n_bits=10  bin_pt=0  load_pin=off  rst=on  en=off  explicit_period=off  period=1  use_behavioral_HDL=off  implementation=Fabric  dbl_ovrd=off  block_type=counter
  ROM : xbsIndex_r4/ROM  depth=1024  initVector=[0:-1:-1024/2+1, 1024/2:-1:1]*(12.8e6/(1024*4))  distributed_mem=Block RAM  rst=off  init_reg=0  en=off  latency=1  gui_display_data_type=Fixed-point  arith_type="Signed  (2's comp)"  n_bits=32  bin_pt=32-ceil(log2(12.8e6/8))-1  preci_type=Single  exp_width=8  frac_width=24  optimize=Area  use_rpm=on  dbl_ovrd=off  simulation_type=fast_sim  block_type=sprom
  Register : xbsIndex_r4/Register  init=0  rst=off  en=on  dbl_ovrd=off  block_type=register
  Register1 : xbsIndex_r4/Register  init=0  rst=off  en=on  dbl_ovrd=off  block_type=register
  Register2 : xbsIndex_r4/Register  init=0  rst=off  en=off  dbl_ovrd=off  block_type=register
  Register3 : xbsIndex_r4/Register  init=0  rst=off  en=off  dbl_ovrd=off  block_type=register
  Register4 : xbsIndex_r4/Register  init=0  rst=on  en=on  dbl_ovrd=off  block_type=register
  Relational : xbsIndex_r4/Relational  mode=a=b  op_type=Bool  en=off  latency=0  dbl_ovrd=off  block_type=relational
  Relational2 : xbsIndex_r4/Relational  mode=a>b  op_type=Bool  en=off  latency=0  dbl_ovrd=off  block_type=relational
  Offset Out : Outport  VectorParamsAs1DForOutWhenUnconnected=off
  wires:
  Register3/1 -> Register4/1, Relational2/1
  SoF/1 -> Counter/1
  Counter/1 -> Relational/2, Register/1
  Constant/1 -> Relational/1
  Relational/1 -> Register2/1, Register4/2
  Register4/1 -> Relational2/2
  Relational2/1 -> Register/2, Register4/3
  Register/1 -> Register1/1
  Register2/1 -> Register1/2
  Register1/1 -> ROM/1
  ROM/1 -> Offset Out/1
  Mag In/1 -> Register3/1

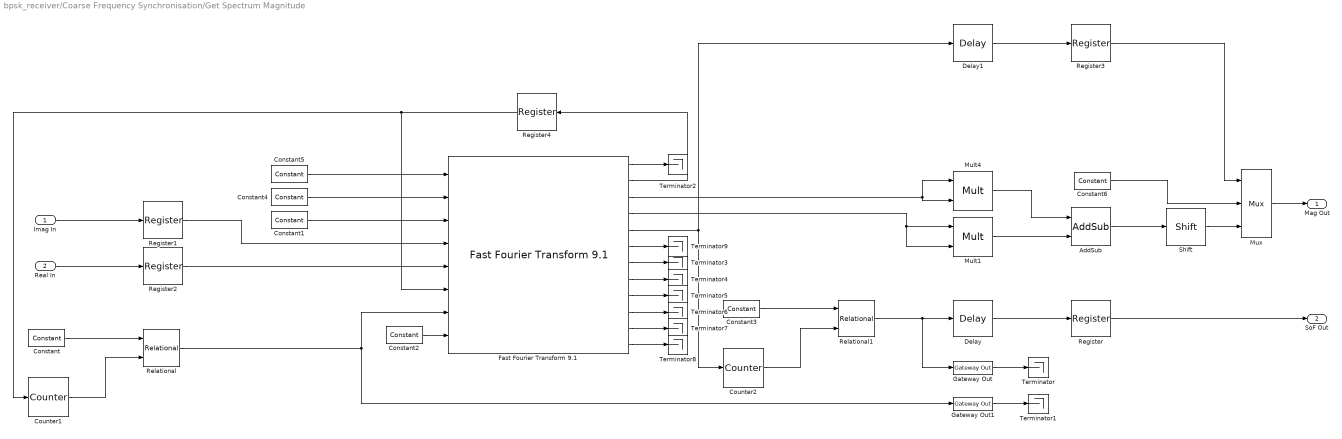
== system bpsk_receiver/Coarse Frequency Synchronisation/Get Spectrum Magnitude ==
  Imag In : Inport
  Real In : Inport  Port=2
  AddSub : xbsIndex_r4/AddSub  mode=Addition  use_carryin=off  use_carryout=off  en=off  latency=1  precision=Full  arith_type=Unsigned  n_bits=16  bin_pt=14  quantization=Truncate  overflow=Wrap  use_behavioral_HDL=off  hw_selection=Fabric  pipelined=off  dbl_ovrd=off  block_type=addsub
  Constant : xbsIndex_r4/Constant  const=1023  gui_display_data_type=Fixed-point  arith_type=Unsigned  n_bits=10  bin_pt=0  preci_type=Single  exp_width=8  frac_width=24  explicit_period=on  period=1/12.8e6  equ=P=C  opselect=C  inp2=PCIN>>17  opr=+  inp1=P  carry=CIN  dbl_ovrd=off  block_type=constant
  Constant1 : xbsIndex_r4/Constant  const=0  gui_display_data_type=Boolean  arith_type=Boolean  n_bits=16  bin_pt=14  preci_type=Single  exp_width=8  frac_width=24  explicit_period=on  period=1/12.8e6  equ=P=C  opselect=C  inp2=PCIN>>17  opr=+  inp1=P  carry=CIN  dbl_ovrd=off  block_type=constant
  Constant2 : xbsIndex_r4/Constant  const=1  gui_display_data_type=Boolean  arith_type=Boolean  n_bits=16  bin_pt=14  preci_type=Single  exp_width=8  frac_width=24  explicit_period=on  period=1/12.8e6  equ=P=C  opselect=C  inp2=PCIN>>17  opr=+  inp1=P  carry=CIN  dbl_ovrd=off  block_type=constant
  Constant3 : xbsIndex_r4/Constant  const=0  gui_display_data_type=Fixed-point  arith_type=Unsigned  n_bits=10  bin_pt=0  preci_type=Single  exp_width=8  frac_width=24  explicit_period=on  period=1/12.8e6  equ=P=C  opselect=C  inp2=PCIN>>17  opr=+  inp1=P  carry=CIN  dbl_ovrd=off  block_type=constant
  Constant4 : xbsIndex_r4/Constant  const=0  gui_display_data_type=Fixed-point  arith_type=Unsigned  n_bits=1  bin_pt=0  preci_type=Single  exp_width=8  frac_width=24  explicit_period=on  period=1/12.8e6  equ=P=C  opselect=C  inp2=PCIN>>17  opr=+  inp1=P  carry=CIN  dbl_ovrd=off  block_type=constant
  Constant5 : xbsIndex_r4/Constant  const=0  gui_display_data_type=Fixed-point  arith_type=Unsigned  n_bits=10  bin_pt=0  preci_type=Single  exp_width=8  frac_width=24  explicit_period=on  period=1/12.8e6  equ=P=C  opselect=C  inp2=PCIN>>17  opr=+  inp1=P  carry=CIN  dbl_ovrd=off  block_type=constant
  Constant6 : xbsIndex_r4/Constant  const=0  gui_display_data_type=Fixed-point  arith_type=Unsigned  n_bits=32  bin_pt=31  preci_type=Single  exp_width=8  frac_width=24  explicit_period=on  period=1/12.8e6  equ=P=C  opselect=C  inp2=PCIN>>17  opr=+  inp1=P  carry=CIN  dbl_ovrd=off  block_type=constant
  Counter1 : xbsIndex_r4/Counter  cnt_type=Count Limited  cnt_to=1023  operation=Up  start_count=0  cnt_by_val=1  arith_type=Unsigned  n_bits=10  bin_pt=0  load_pin=off  rst=off  en=on  explicit_period=on  period=1/12.8e6  use_behavioral_HDL=off  implementation=Fabric  dbl_ovrd=off  block_type=counter
  Counter2 : xbsIndex_r4/Counter  cnt_type=Count Limited  cnt_to=1023  operation=Up  start_count=0  cnt_by_val=1  arith_type=Unsigned  n_bits=10  bin_pt=0  load_pin=off  rst=off  en=on  explicit_period=on  period=1/12.8e6  use_behavioral_HDL=off  implementation=Fabric  dbl_ovrd=off  block_type=counter
  Delay : xbsIndex_r4/Delay  rst=off  infoeditControl=Selection of Reset will increase slice count due to use of real FFs and instead of SRLs  en=off  latency=3  reg_retiming=off  dbl_ovrd=off  block_type=delay
  Delay1 : xbsIndex_r4/Delay  rst=off  infoeditControl=Selection of Reset will increase slice count due to use of real FFs and instead of SRLs  en=off  latency=3  reg_retiming=off  dbl_ovrd=off  block_type=delay
  "Fast Fourier Transform 9.1 " : xbsIndex_r4/Fast Fourier Transform 9.1   transform_length=1024  target_clock_frequency=128  target_data_throughput=13  implementation_options=pipelined_streaming_io  run_time_configurable_transform_length=off  phase_factor_width=16  scaling_options=scaled  rounding_modes=truncation  aclken=off  aresetn=off  output_ordering=natural_order  cyclic_prefix_insertion=off  throttle_scheme=nonrealtime  xk_index=off  ovflo=off  trim_axipin_name=on  memory_options_data=block_ram  memory_options_phase_factors=block_ram  number_of_stages_using_block_ram_for_data_and_phase_factors=1  memory_options_reorder=block_ram  memory_options_hybrid=off  complex_mult_type=use_mults_resources  butterfly_type=use_luts  simulation_type=hybrid_sim  simulation_model=sysgen:xfftv9_cmodel  data_path_portlist={ 's_axis_data_tdata', 'm_axis_data_tdata', 'm_axis_status_tdata', 'event_fft_overflow' }  channels=1  input_ordering=natural_order  input_width=16  ip_name=Fast Fourier Transform  ip_version=9.1  dsptool_ready=true  ipcore_usecache=true  ipcore_useipmodelcache=true  wrapper_available=true  port_translation_map={ 'aclken' => 'en', 'aresetn' => 'rst'}  data_format=fixed_point  block_type=xfft_v9_1
  Gateway Out : xbsIndex_r4/Gateway Out  inherit_from_input=on  hdl_port=off  rows=1  columns=1  UseAsDAC=off  DACChannel='1'  interface=None  automatic_assignment=on  address_offset=hex2dec('00')  intf_name=''  intf_description=''  timing_constraint=None  locs_specified=off  LOCs={}  io_standard={}  block_type=gatewayout
  Gateway Out1 : xbsIndex_r4/Gateway Out  inherit_from_input=on  hdl_port=off  rows=1  columns=1  UseAsDAC=off  DACChannel='1'  interface=None  automatic_assignment=on  address_offset=hex2dec('00')  intf_name=''  intf_description=''  timing_constraint=None  locs_specified=off  LOCs={}  io_standard={}  block_type=gatewayout
  Mult1 : xbsIndex_r4/Mult  precision=User Defined  arith_type=Unsigned  n_bits=63  bin_pt=62  quantization=Truncate  overflow=Saturate  en=off  latency=3  use_behavioral_HDL=off  opt=Speed  use_embedded=on  optimum_pipeline=off  pipeline=on  dbl_ovrd=off  use_rpm=on  placement_style=Triangular  block_type=mult
  Mult4 : xbsIndex_r4/Mult  precision=User Defined  arith_type=Unsigned  n_bits=63  bin_pt=62  quantization=Truncate  overflow=Saturate  en=off  latency=3  use_behavioral_HDL=off  opt=Speed  use_embedded=on  optimum_pipeline=off  pipeline=on  dbl_ovrd=off  use_rpm=on  placement_style=Triangular  block_type=mult
  Mux : xbsIndex_r4/Mux  inputs=2  en=off  latency=0  precision=Full  arith_type=Unsigned  n_bits=16  bin_pt=14  quantization=Truncate  overflow=Wrap  dbl_ovrd=off  block_type=mux
  Register{,1..4} (5 alike) : xbsIndex_r4/Register  init=0  rst=off  en=off  dbl_ovrd=off  block_type=register
  Relational : xbsIndex_r4/Relational  mode=a=b  op_type=Bool  en=off  latency=0  dbl_ovrd=off  block_type=relational
  Relational1 : xbsIndex_r4/Relational  mode=a=b  op_type=Bool  en=off  latency=0  dbl_ovrd=off  block_type=relational
  Shift : xbsIndex_r4/Shift  shift_dir=Right  shift_bits=2  en=off  latency=0  precision=User Defined  arith_type=Unsigned  n_bits=32  bin_pt=31  quantization=Truncate  overflow=Wrap  dbl_ovrd=off  block_type=shift
  Terminator{,1..9} (10 alike) : Terminator
  Mag Out : Outport  VectorParamsAs1DForOutWhenUnconnected=off
  SoF Out : Outport  Port=2  VectorParamsAs1DForOutWhenUnconnected=off
  wires:
  Register3/1 -> Mux/1
  Delay1/1 -> Register3/1
  Constant6/1 -> Mux/2
  Shift/1 -> Mux/3
  Mux/1 -> Mag Out/1
  Constant5/1 -> "Fast Fourier Transform 9.1 "/1
  Constant4/1 -> "Fast Fourier Transform 9.1 "/2
  "Fast Fourier Transform 9.1 "/6 -> Terminator9/1
  "Fast Fourier Transform 9.1 "/5 -> Delay1/1, Counter2/1
  Constant3/1 -> Relational1/1
  Counter2/1 -> Relational1/2
  "Fast Fourier Transform 9.1 "/12 -> Terminator8/1
  "Fast Fourier Transform 9.1 "/11 -> Terminator7/1
  "Fast Fourier Transform 9.1 "/10 -> Terminator6/1
  "Fast Fourier Transform 9.1 "/9 -> Terminator5/1
  "Fast Fourier Transform 9.1 "/8 -> Terminator4/1
  "Fast Fourier Transform 9.1 "/7 -> Terminator3/1
  Constant1/1 -> "Fast Fourier Transform 9.1 "/3
  "Fast Fourier Transform 9.1 "/1 -> Terminator2/1
  Counter1/1 -> Relational/2
  Gateway Out1/1 -> Terminator1/1
  Gateway Out/1 -> Terminator/1
  Relational/1 -> Gateway Out1/1, "Fast Fourier Transform 9.1 "/7
  Constant/1 -> Relational/1
  Relational1/1 -> Delay/1, Gateway Out/1
  "Fast Fourier Transform 9.1 "/4 -> Mult1/2, Mult1/1
  Real In/1 -> Register2/1
  "Fast Fourier Transform 9.1 "/3 -> Mult4/2, Mult4/1
  Imag In/1 -> Register1/1
  Delay/1 -> Register/1
  Register/1 -> SoF Out/1
  Register1/1 -> "Fast Fourier Transform 9.1 "/4
  Register2/1 -> "Fast Fourier Transform 9.1 "/5
  Mult1/1 -> AddSub/2
  Mult4/1 -> AddSub/1
  AddSub/1 -> Shift/1
  Register4/1 -> Counter1/1, "Fast Fourier Transform 9.1 "/6
  "Fast Fourier Transform 9.1 "/2 -> Register4/1
  Constant2/1 -> "Fast Fourier Transform 9.1 "/8

== system bpsk_receiver/Coarse Frequency Synchronisation/Increase Signal Power ==
  note: 18-bit multiply for DSP48E2
  note: Product block is required as it is a complex multiplication
  Imag In : Inport
  Real In : Inport  Port=2
  Convert : xbsIndex_r4/Convert  gui_display_data_type=Fixed-point  arith_type="Signed  (2's comp)"  n_bits=32  bin_pt=31  float_type=Single  exp_bits=8  fraction_bits=24  quantization=Truncate  overflow=Wrap  en=off  latency=0  pipeline=off  dbl_ovrd=off  block_type=convert
  Convert1 : xbsIndex_r4/Convert  gui_display_data_type=Fixed-point  arith_type="Signed  (2's comp)"  n_bits=32  bin_pt=31  float_type=Single  exp_bits=8  fraction_bits=24  quantization=Truncate  overflow=Wrap  en=off  latency=0  pipeline=off  dbl_ovrd=off  block_type=convert
  Convert2 : xbsIndex_r4/Convert  gui_display_data_type=Fixed-point  arith_type="Signed  (2's comp)"  n_bits=18  bin_pt=15  float_type=Single  exp_bits=8  fraction_bits=24  quantization=Truncate  overflow=Wrap  en=off  latency=0  pipeline=off  dbl_ovrd=off  block_type=convert
  Convert4 : xbsIndex_r4/Convert  gui_display_data_type=Fixed-point  arith_type="Signed  (2's comp)"  n_bits=18  bin_pt=15  float_type=Single  exp_bits=8  fraction_bits=24  quantization=Truncate  overflow=Wrap  en=off  latency=0  pipeline=off  dbl_ovrd=off  block_type=convert
  Product1 : xbsIndex_r4/Product  complex_multiplier=on  optimizegoal=Performance  simulation_type=fast_sim  simulation_model=sysgen:product_macro  block_type=product_macro
  Product2 : xbsIndex_r4/Product  complex_multiplier=on  optimizegoal=Performance  simulation_type=fast_sim  simulation_model=sysgen:product_macro  block_type=product_macro
  Imag Out : Outport  VectorParamsAs1DForOutWhenUnconnected=off
  Real Out : Outport  Port=2  VectorParamsAs1DForOutWhenUnconnected=off
  wires:
  Imag In/1 -> Product2/2, Product2/4
  Real In/1 -> Product2/1, Product2/3
  Product2/1 -> Convert4/1
  Product2/2 -> Convert2/1
  Convert4/1 -> Product1/1, Product1/3
  Convert2/1 -> Product1/4, Product1/2
  Product1/1 -> Convert/1
  Product1/2 -> Convert1/1
  Convert/1 -> Real Out/1
  Convert1/1 -> Imag Out/1
